simulink model "furuta_pendulum_response_feedback_c"  (R2016a)
settings: Solver=VariableStepAuto  StartTime=0.0  StopTime=40  MaxStep=1e-3  RelTol=1e-3
undefined symbols (not defined in the file): L
settings Model: Creator=mgreiff  LastModifiedBy=mgreiff

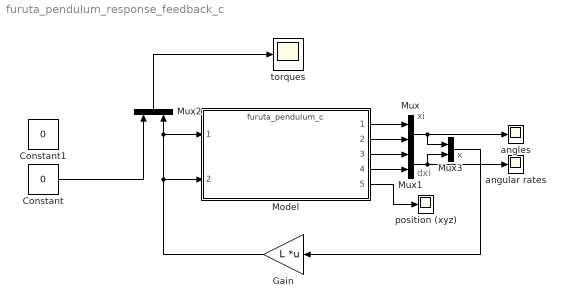
== system furuta_pendulum_response_feedback_c ==
  note: dxi
  note: xi
  note: x
  Constant : Constant  Value=0
  Constant1 : Constant  Value=0
  Gain : Gain  Gain=L  Multiplication=Matrix(K*u)
  Model : ModelReference  ModelNameDialog=furuta_pendulum_c.slx  SimulationMode=Normal  ModelReferenceVersion=1.32
  Mux{,1..3} (4 alike) : Mux  Inputs=2
  angles : Scope
  angular rates : Scope
  position (xyz) : Scope
  torques : Scope
  wires:
  Model/1 -> Mux/1
  Model/3 -> Mux1/1
  Model/4 -> Mux1/2
  Mux1/1 -> angular rates/1, Mux3/2
  Model/2 -> Mux/2
  Mux/1 -> Mux3/1, angles/1
  Mux2/1 -> torques/1
  Mux3/1 -> Gain/1
  Model/5 -> position (xyz)/1
  Constant/1 -> Mux2/1
  Gain/1 -> Model/2, Mux2/2, Model/1
